simulink model "EjemploServidorM2011b"  (Simulink 7.8)
settings: Solver=ode3  StartTime=0.0  StopTime=inf  FixedStep=0.001  RelTol=1e-3
libraries: aerolibanimutils x1
settings Model: Creator=Usuario  LastModifiedBy=Sebastián
settings OptimizationCC: SimCompilerOptimization=On
settings CodeAppCC: CustomSymbolStrType=$N$R$M_T

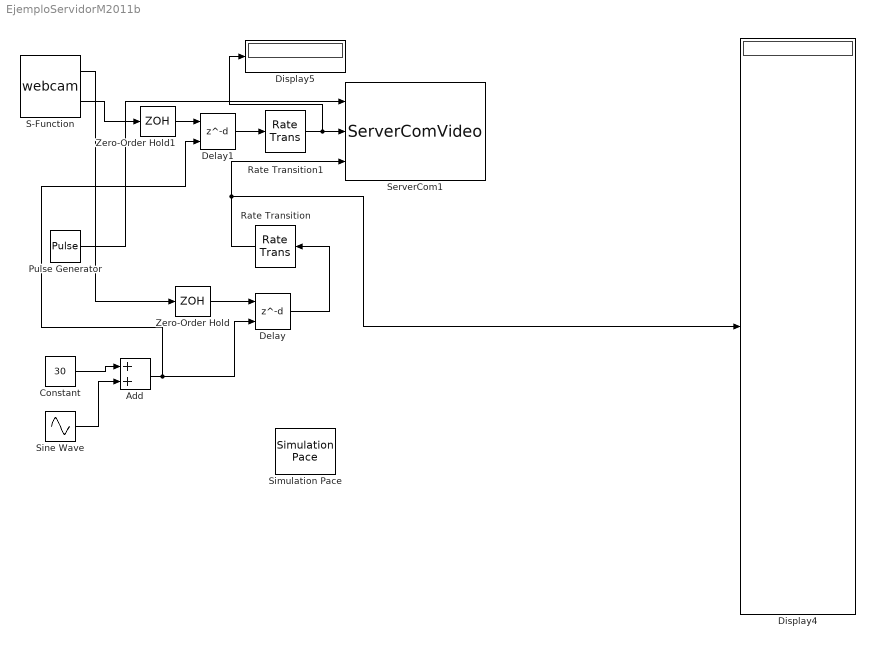
== system EjemploServidorM2011b ==
  Add : Sum  SampleTime=0.05
  Constant : Constant  Value=30  SampleTime=0.05
  Delay : Delay  DelayLengthSource=Input port  SampleTime=0.05
      settings: InputPortMap=u0,p1
  Delay1 : Delay  DelayLengthSource=Input port  SampleTime=0.05
      settings: InputPortMap=u0,p1
  Display4 : Display
  Display5 : Display
  Pulse Generator : DiscretePulseGenerator  PulseType=Time based  Period=0.05  PulseWidth=50
  Rate Transition : RateTransition  OutPortSampleTime=0
  Rate Transition1 : RateTransition  OutPortSampleTime=0
  S-Function : S-Function  FunctionName=webcam  Parameters=1  EnableBusSupport=off
  ServerCom1 : S-Function  FunctionName=ServerComVideo  EnableBusSupport=off
      mask Display:
      | patch([0 4. 4 0],[0.02 0.02 0.98 0.98],0.9*[123 193 255]/255)
      | patch([0 4 4 0],[0.1 0.1 0.9 0.9],[123 193 255]/255)
      | patch([1.5 2.5 2.5 2.3 2.3 1.7 1.7 1.5],[0 0 1 1 1.2 1.2 1 1],[130 130 130]/255)
      | patch([1.3 2.7 2.7 1.3],[1.2 1.2 2.9 2.9],0.85*[130 130 130]/255)
      | patch([1.4 2.6 2.6 1.4],[1.3 1.3 2.8 2.8],[123 193 255]/255)
      | patch([1.5 2.5 2.5 1.5],[1.4 1.4 2.7 2.7],0.85*[130 130 130]/255)
      | patch([1.9 2.1 2.1 1.9],[1.8 1.8 2.1 2.1],[123 193 255]/255)
      | color('red')
      | port_label('input',1,'clock')
      | port_label('input',2,'sizeSend')
      | port_label('input',3,'dataSend')
      | port_label('output',1,'stateChannel')
      | port_label('output',2,'dataRecv')
  Simulation Pace : aerolibanimutils/Simulation Pace  SimulationPace=1  SleepMode=MATLAB Thread  OutputPaceError=off  SampleTime=-1
      settings: AttributesFormatString=%<SimulationPace> sec/sec
  Sine Wave : Sin  Amplitude=10  Frequency=0.1*2*pi  SampleTime=0.05
  Zero-Order Hold : ZeroOrderHold  SampleTime=0.05
  Zero-Order Hold1 : ZeroOrderHold  SampleTime=0.05
  wires:
  Pulse Generator/1 -> ServerCom1/1
  S-Function/2 -> Zero-Order Hold1/1
  Zero-Order Hold/1 -> Delay/1
  Sine Wave/1 -> Add/2
  Constant/1 -> Add/1
  Add/1 -> Delay1/2, Delay/2
  Delay/1 -> Rate Transition/1
  S-Function/1 -> Zero-Order Hold/1
  Rate Transition/1 -> Display4/1, ServerCom1/3
  Delay1/1 -> Rate Transition1/1
  Rate Transition1/1 -> Display5/1, ServerCom1/2
  Zero-Order Hold1/1 -> Delay1/1
